simulink model "DensityComputation"  (R2025a)
settings: Solver=ode23tb  StartTime=0.0  StopTime=1000  MaxStep=0.1  RelTol=1e-3
undefined symbols (not defined in the file): DENSITY_BIAS, DENSITY_MODEL_A, DENSITY_MODEL_B
settings Model: DataDictionary=FuelGaugingData.sldd  Creator=mkelley  LastModifiedBy=mkelley

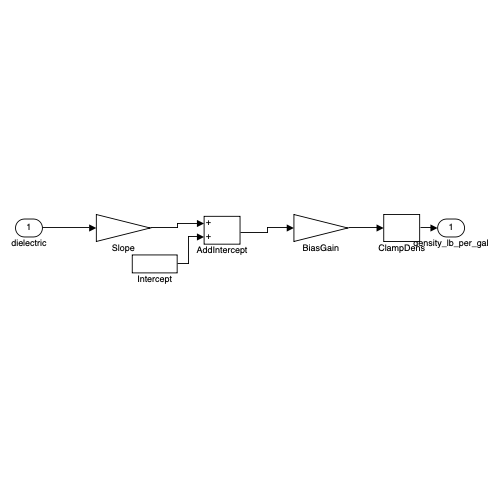
[thumbnail: Simulink's stored preview of the top-level diagram]
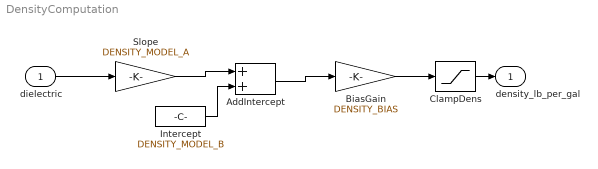
== system DensityComputation ==
  dielectric : Inport
  AddIntercept : Sum
  BiasGain : Gain  Gain=DENSITY_BIAS
  ClampDens : Saturate  UpperLimit=8.5  LowerLimit=5.5
  Intercept : Constant  Value=DENSITY_MODEL_B
  Slope : Gain  Gain=DENSITY_MODEL_A
  density_lb_per_gal : Outport
  wires:
  dielectric/1 -> Slope/1
  Slope/1 -> AddIntercept/1
  Intercept/1 -> AddIntercept/2
  AddIntercept/1 -> BiasGain/1
  BiasGain/1 -> ClampDens/1
  ClampDens/1 -> density_lb_per_gal/1
